simulink model "dz_3_simul_model"  (R2026a)
settings: Solver=VariableStepAuto  StopTime=30
values from neighbouring files (symbols this model uses):
  g = 9.81    [dz_3_model.m]
  mass_quadrotor = 1.07    [dz_3_model.m]
settings Model: Creator=vas77  LastModifiedBy=vas77
settings HardwareCC: ProdHWDeviceType=AMD->x86-64 (Windows64)
settings RTWCC: BuildConfiguration=Faster Runs

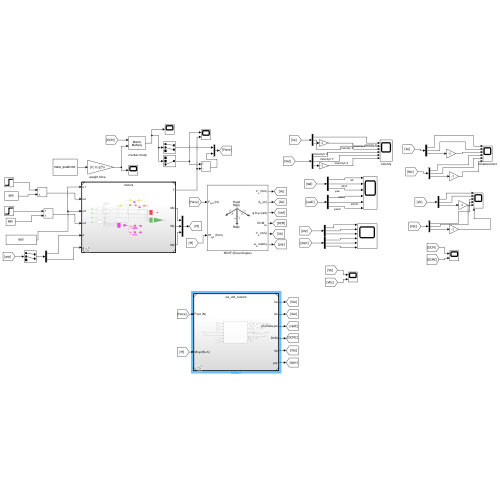
[thumbnail: Simulink's stored preview of the top-level diagram]
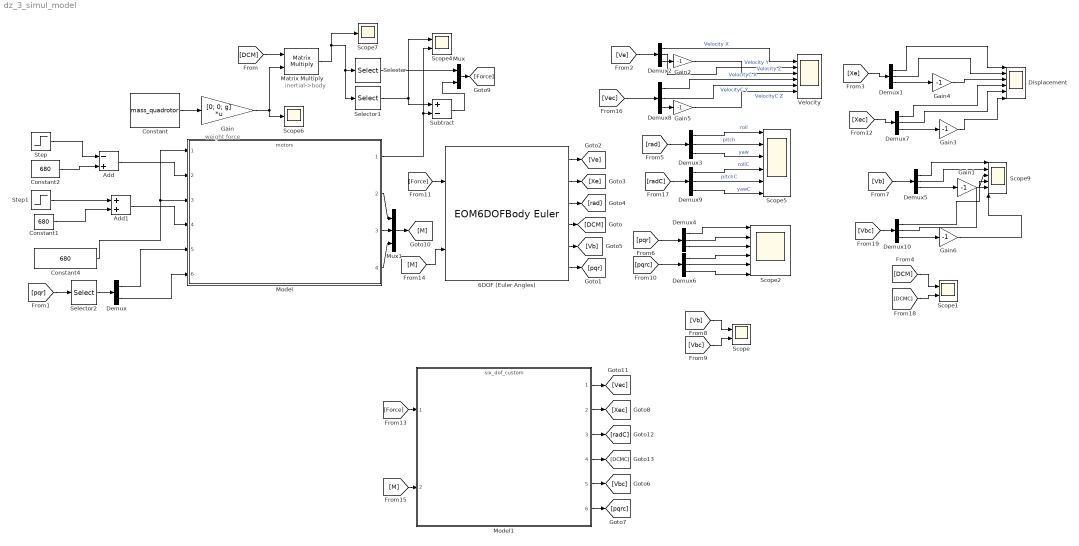
== system dz_3_simul_model ==
  note: weight force
  note: inertial->body
  6DOF (Euler Angles) : EOM6DOFBodyEuler  mass_0=mass_quadrotor  inertia=I
  Add : Sum  Inputs=-+
  Add1 : Sum
  Constant : Constant  Value=mass_quadrotor  VectorParams1D=off
  Constant1 : Constant  Value=680
  Constant2 : Constant  Value=680
  Constant4 : Constant  Value=680
  Demux : Demux  Outputs=2
  Demux{1..10} (10 alike) : Demux  Outputs=3
  Displacement : Scope  NumInputPorts=6
      settings: Title=Displacement X (m)  ActiveDisplayYMinimum=-27.785695670857422  ActiveDisplayYMaximum=250.07126103771685  YLabel=Displacement X (m)  DataLoggingVariableName=ScopeData8
  Gain : Gain  Gain=[0; 0; g]  Multiplication=Matrix(K*u)
  Gain{1..6} (6 alike) : Gain  Gain=-1
  Matrix Multiply : Product  Multiplication=Matrix(*)
  Model : ModelReference  ModelNameDialog=motors.slx  SimulationMode=Normal  ModelReferenceVersion=1.19
  Model1 : ModelReference  ModelNameDialog=six_dof_custom.slx  SimulationMode=Normal  ModelReferenceVersion=1.11
  Mux : Mux  Inputs=2
  Mux1 : Mux  Inputs=3
  Scope : Scope  NumInputPorts=2
      settings: ActiveDisplayYMinimum=-290.57421233945433  ActiveDisplayYMaximum=293.89722140345123  DataLoggingVariableName=ScopeData9
  Scope1 : Scope  NumInputPorts=2
      settings: ActiveDisplayYMinimum=-1.24988698292059  ActiveDisplayYMaximum=1.2499874425467321
  Scope2 : Scope  NumInputPorts=6
      settings: ActiveDisplayYMinimum=-33.808125357697485  ActiveDisplayYMaximum=33.826743561939026  DataLoggingVariableName=ScopeData2
  Scope4 : Scope  NumInputPorts=2
      settings: ActiveDisplayYMinimum=5.9584764482034869  ActiveDisplayYMaximum=15.675635410083268  DataLoggingVariableName=ScopeData4
  Scope5 : Scope  NumInputPorts=6
      settings: Title=Roll, pitch, yaw  ActiveDisplayYMinimum=-3.9265875675420774  ActiveDisplayYMaximum=3.9251981526870274  YLabel=Roll, pitch, yaw( rad )  DataLoggingVariableName=ScopeData3
  Scope6 : Scope
      settings: ActiveDisplayYMinimum=5.1775949245841977  ActiveDisplayYMaximum=10.902189225640303  DataLoggingVariableName=ScopeData6
  Scope7 : Scope
      settings: ActiveDisplayYMinimum=-1  ActiveDisplayYMaximum=1  DataLoggingVariableName=ScopeData7
  Scope9 : Scope  NumInputPorts=6
      settings: ActiveDisplayString=3  Title=Velocity Z  ActiveDisplayYMinimum=-293.60589191209095  ActiveDisplayYMaximum=290.54184239596987  YLabel=Speed(m/s)  DataLoggingVariableName=ScopeData5
  Selector : Selector  IndexMode=Zero-based  InputPortWidth=3  IndexOptions=Index vector (dialog)  Indices=[0 1]  OutputSizes=1
  Selector1 : Selector  IndexMode=Zero-based  InputPortWidth=3  IndexOptions=Index vector (dialog)  Indices=[2]  OutputSizes=1
  Selector2 : Selector  IndexMode=Zero-based  InputPortWidth=3  IndexOptions=Index vector (dialog)  Indices=[0 1]  OutputSizes=1
  Step : Step  Time=4  FinalValue=10  SampleTime=0
  Step1 : Step  Time=4  FinalValue=10  SampleTime=0
  Subtract : Sum  Inputs=+-
  Velocity : Scope  NumInputPorts=6
      settings: Title=Velocity ( Earth )  ActiveDisplayYMinimum=-2.4170261786507035  ActiveDisplayYMaximum=21.753235607856336  YLabel=Speed(m/s)
  wires:
  Constant/1 -> Gain/1
  [DCM] -> Matrix Multiply/1
  Gain/1 -> Matrix Multiply/2, Scope6/1
  Matrix Multiply/1 -> Scope7/1, Selector1/1, Selector/1
  Selector1/1 -> Scope4/1, Subtract/1
  Subtract/1 -> Mux/2
  Selector/1 -> Mux/1
  Model/1 -> Scope4/2, Subtract/2
  Model/2 -> Mux1/1
  Model/3 -> Mux1/2
  Model/4 -> Mux1/3
  6DOF (Euler Angles)/4 -> [DCM]
  [pqr] -> Selector2/1
  Demux/1 -> Model/5
  Demux/2 -> Model/6
  Selector2/1 -> Demux/1
  6DOF (Euler Angles)/2 -> [Xe]
  Demux1/1 -> Displacement/1
  Demux1/2 -> Displacement/2
  Demux1/3 -> Gain4/1
  Gain4/1 -> Displacement/3
  6DOF (Euler Angles)/1 -> [Ve]
  Demux2/3 -> Gain2/1
  Gain2/1 -> Velocity/3  "Velocity Z"
  Demux2/2 -> Velocity/2  "Velocity Y"
  Demux2/1 -> Velocity/1  "Velocity X"
  [DCM] -> Scope1/1
  [rad] -> Demux3/1
  Demux3/2 -> Scope5/2  "pitch"
  Demux3/1 -> Scope5/1  "roll"
  6DOF (Euler Angles)/3 -> [rad]
  6DOF (Euler Angles)/6 -> [pqr]
  Demux3/3 -> Scope5/3  "yaw"
  [pqr] -> Demux4/1
  Demux4/2 -> Scope2/2
  Demux4/3 -> Scope2/3
  Demux4/1 -> Scope2/1
  [Ve] -> Demux2/1
  [Xe] -> Demux1/1
  [Vb] -> Demux5/1
  Demux5/1 -> Scope9/1
  Demux5/2 -> Scope9/2
  Gain1/1 -> Scope9/3
  Demux5/3 -> Gain1/1
  6DOF (Euler Angles)/5 -> [Vb]
  Step/1 -> Add/1
  Constant2/1 -> Add/2
  Constant1/1 -> Add1/2
  Step1/1 -> Add1/1
  Constant4/1 -> Model/3, Model/1
  Add/1 -> Model/2
  Add1/1 -> Model/4
  [Vb] -> Scope/1
  [Vbc] -> Scope/2
  Demux6/1 -> Scope2/4
  Demux6/2 -> Scope2/5
  [pqrc] -> Demux6/1
  Demux6/3 -> Scope2/6
  Demux7/2 -> Displacement/5
  Demux7/1 -> Displacement/4
  Demux7/3 -> Gain3/1
  [Xec] -> Demux7/1
  Gain3/1 -> Displacement/6
  [Force] -> 6DOF (Euler Angles)/1
  Mux/1 -> [Force]
  [Force] -> Model1/1
  Mux1/1 -> [M]
  [M] -> 6DOF (Euler Angles)/2
  [M] -> Model1/2
  Model1/2 -> [Xec]
  Model1/1 -> [Vec]
  Gain5/1 -> Velocity/6  "VelocityC Z"
  [Vec] -> Demux8/1
  Demux8/1 -> Velocity/4  "VelocityC X"
  Demux8/3 -> Gain5/1
  Demux8/2 -> Velocity/5  "VelocityC Y"
  Model1/6 -> [pqrc]
  Model1/5 -> [Vbc]
  Model1/3 -> [radC]
  Model1/4 -> [DCMC]
  [DCMC] -> Scope1/2
  [radC] -> Demux9/1
  Demux9/1 -> Scope5/4  "rollC"
  Demux9/3 -> Scope5/6  "yawC"
  Demux9/2 -> Scope5/5  "pitchC"
  Demux10/1 -> Scope9/4
  Demux10/2 -> Scope9/5
  Gain6/1 -> Scope9/6
  Demux10/3 -> Gain6/1
  [Vbc] -> Demux10/1
